simulink model "tisch"  (R2015a)
settings: Solver=ode45  SolverMode=SingleTasking  StartTime=0.0  StopTime=10.0  RelTol=1e-3
settings Model: CovSFcnEnable=off  Creator=john  LastModifiedBy=john
settings OptimizationCC: BlockReduction=off  BooleanDataType=off
settings DebuggingCC: SaveWithParameterizedLinksMsg=none  UnderspecifiedInitializationDetection=Classic  MergeDetectMultiDrivingBlocksExec=none  SignalResolutionControl=TryResolveAllWithWarning
settings HardwareCC: TargetUnknown=on

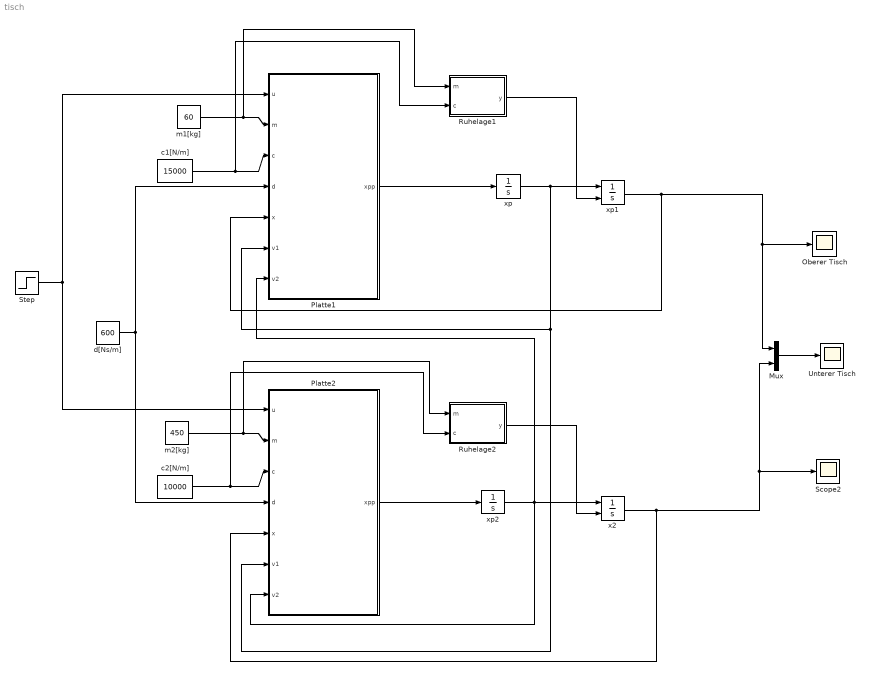
== system tisch ==
  Mux : Mux  Inputs=2
  Oberer Tisch : Scope
  Platte1 : MATLAB Function  TreatAsAtomicUnit=on
  Platte2 : MATLAB Function  TreatAsAtomicUnit=on
  Ruhelage1 : MATLAB Function  TreatAsAtomicUnit=on
  Ruhelage2 : MATLAB Function  TreatAsAtomicUnit=on
  Scope2 : Scope
      settings: SaveName=ScopeData2
  Step : Step  After=0.002  SampleTime=0
  Unterer Tisch : Scope
      settings: TimeRange=10
  c1[N/m] : Constant  Value=15000
  c2[N/m] : Constant  Value=10000
  d[Ns/m] : Constant  Value=600
  m1[kg] : Constant  Value=60
  m2[kg] : Constant  Value=450
  x2 : Integrator  InitialConditionSource=external
  xp : Integrator
  xp1 : Integrator  InitialConditionSource=external
  xp2 : Integrator
  wires:
  Platte1/1(xpp) -> xp/1
  m1[kg]/1 -> Ruhelage1/1(m), Platte1/2(m)
  c1[N/m]/1 -> Ruhelage1/2(c), Platte1/3(c)
  d[Ns/m]/1 -> Platte2/4(d), Platte1/4(d)
  xp/1 -> xp1/1, Platte2/6(v1), Platte1/6(v1)
  Platte2/1(xpp) -> xp2/1
  xp2/1 -> Platte1/7(v2), x2/1, Platte2/7(v2)
  x2/1 -> Scope2/1, Mux/2, Platte2/5(x)
  xp1/1 -> Oberer Tisch/1, Mux/1, Platte1/5(x)
  c2[N/m]/1 -> Ruhelage2/2(c), Platte2/3(c)
  m2[kg]/1 -> Ruhelage2/1(m), Platte2/2(m)
  Mux/1 -> Unterer Tisch/1
  Step/1 -> Platte1/1(u), Platte2/1(u)
  Ruhelage1/1(y) -> xp1/2
  Ruhelage2/1(y) -> x2/2

== matlab function tisch/Platte2 ==
  data: u input; xpp output; m input; c input; d input; x input; v1 input; v2 input
function xpp = fcn(u, m, c, d, x, v1, v2)

g = 9.81;

FG = (m * g);
FF = -1 * (c * ((x - u)));
FD = (d * (v1 + v2));

xpp = (2 * (FF - FD) - FG) / m;

== matlab function tisch/Platte1 ==
  data: u input; xpp output; m input; c input; d input; x input; v1 input; v2 input
function xpp = fcn(u, m, c, d, x, v1, v2)

g = 9.81;

FG = (m * g);
FF = -1 * (c * ((x - u)));
FD = (d * (v1 + v2));

xpp = (2 * (FF - FD) - FG) / m;

== matlab function tisch/Ruhelage1 ==
  data: m input; y output; c input
function y = fcn(m, c)
%#codegen

g = 9.81;

FG = m * g;

y = -1 * ((FG / (2 * c)));

== matlab function tisch/Ruhelage2 ==
  data: m input; y output; c input
function y = fcn(m, c)
%#codegen

g = 9.81;

FG = m * g;

y = -1 * ((FG / (2 * c)));
